simulink model "FM_Nuand_RX"  (R2022b)
settings: Solver=FixedStepAuto  StartTime=0.0  StopTime=inf  RelTol=1e-3
libraries: dspsnks4 x1, dspsigops x1, commanabbnd3 x1
settings Model: Creator=Gitub  LastModifiedBy=Gitub

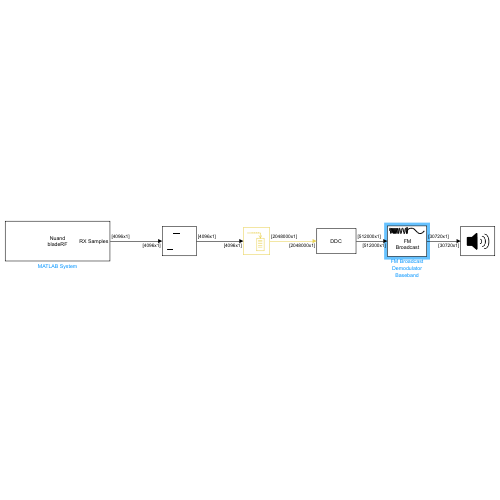
[thumbnail: Simulink's stored preview of the top-level diagram]
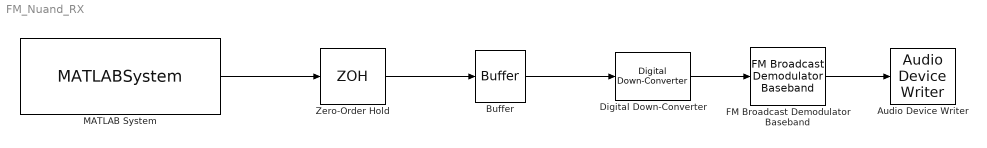
== system FM_Nuand_RX ==
  Audio Device Writer : dspsnks4/Audio Device Writer  Driver=DirectSound  Device=Default  InheritSampleRate=off  SampleRate=48e3  BitDepth=16-bit integer  BufferSize=4096  NumBuffers=10  DefaultOutputChannelMapping=on  OutputChannelMapping=1:2  OutputNumUnderrunSamples=off  DriverIdx=1  DeviceWarnFlag=Altavoces (JBL GO 2 Stereo)
  Buffer : Buffer  N=4096*500  OutputFrames=off
  Digital Down-Converter : dspsigops/Digital Down-Converter  DecimationFactor=4  MinimumOrderDesign=on  NumCICSections=3  ThirdFilterOrder=10  StopbandFrequencySource=Auto  Oscillator=Sine wave  CenterFrequency=0  SecondFilterOrder=12  Bandwidth=0.2e6  StopbandFrequency=150000  PassbandRipple=0.1  StopbandAttenuation=80  NumAccumulatorBits=16  NumQuantizedAccumulatorBits=12  Dither=on  NumDitherBits=4  InheritSampleRate=off  SampleRate=2e6  SimulateUsing=Interpreted execution  outputMin=[]  outputMax=[]
  FM Broadcast Demodulator Baseband : commanabbnd3/FM Broadcast Demodulator Baseband  SampleRate=800e3  FrequencyDeviation=75e3  FilterTimeConstant=75e-6  AudioSampleRate=48e3  PlaySound=off  BufferSize=4096  Stereo=off  RBDS=off  RBDSSamplesPerSymbol=10  RBDSCostasLoop=off  SimulateUsing=Interpreted execution
  MATLAB System : MATLABSystem  System=bladeRF_Simulink  loopback_mode=None  xb200=off  SimulateUsing=Interpreted execution  enable_rx=on  enable_overrun=off  rx_frequency=88.9e6  rx_samplerate=2e6  rx_bandwidth=6  rx_gain=0  enable_rx_biastee=off  rx_agc=AUTO  rx_num_buffers=32  rx_num_transfers=16  rx_buf_size=1024*4  rx_timeout_ms=3000  rx_step_size=1024*4  enable_tx=off  enable_underrun=off  tx_frequency=920e6  tx_samplerate=3e6  tx_bandwidth=20  tx_gain=60  enable_tx_biastee=off  tx_num_buffers=64  tx_num_transfers=16  tx_buf_size=1024  tx_timeout_ms=3000  tx_step_size=1024  verbosity=Info
      mask Type: bladeRF_Simulink
      mask Display:
      | disp(['Nuand' char(10) 'bladeRF']);
      | port_label('output',1,'RX Samples');
  Zero-Order Hold : ZeroOrderHold  SampleTime=1/(4096)
  wires:
  Zero-Order Hold/1 -> Buffer/1
  MATLAB System/1 -> Zero-Order Hold/1
  Buffer/1 -> Digital Down-Converter/1
  Digital Down-Converter/1 -> FM Broadcast Demodulator Baseband/1
  FM Broadcast Demodulator Baseband/1 -> Audio Device Writer/1
